simulink model "BlokSchema2"  (R2022a)
settings: Solver=VariableStepAuto  StartTime=0.0  StopTime=10000  RelTol=1e-3
undefined symbols (not defined in the file): citatel, Delay, Grz_spatnaObdlMet, Grz_tustin, menovatel, T
settings Model: PacingRate=100  Creator=domin  LastModifiedBy=domin
settings ModelReferenceCC: EnableRefExpFcnMdlSchedulingChecks=off
settings RTWCC: Description=Generic Real-Time Target

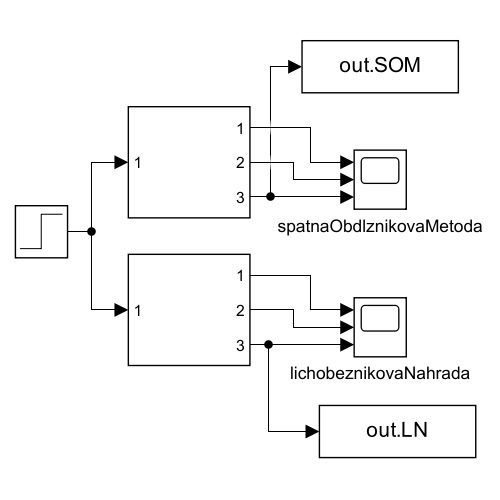
[thumbnail: Simulink's stored preview of the top-level diagram]
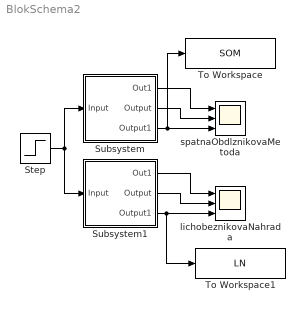
== system BlokSchema2 ==
  Step : Step  Time=0  Before=1  SampleTime=0
  Subsystem : Subsystem
  Subsystem1 : Subsystem
  To Workspace : ToWorkspace  VariableName=SOM  SampleTime=-1
  To Workspace1 : ToWorkspace  VariableName=LN  SampleTime=-1
  lichobeznikovaNahrada : Scope  NumInputPorts=3
  spatnaObdlznikovaMetoda : Scope  NumInputPorts=3
  wires:
  Step/1 -> Subsystem/1(Input), Subsystem1/1(Input)
  Subsystem/1(Out1) -> spatnaObdlznikovaMetoda/1
  Subsystem/2(Output) -> spatnaObdlznikovaMetoda/2
  Subsystem/3(Output1) -> To Workspace/1, spatnaObdlznikovaMetoda/3
  Subsystem1/1(Out1) -> lichobeznikovaNahrada/1
  Subsystem1/2(Output) -> lichobeznikovaNahrada/2
  Subsystem1/3(Output1) -> To Workspace1/1, lichobeznikovaNahrada/3

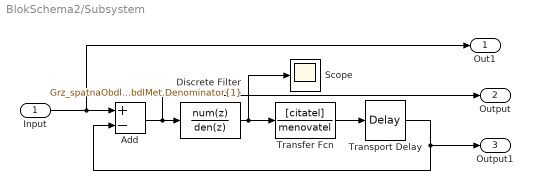
== system BlokSchema2/Subsystem ==
  Input : Inport
  Add : Sum  Inputs=+-
  Discrete Filter : DiscreteFilter  Numerator=Grz_spatnaObdlMet.Numerator{1}  Denominator=Grz_spatnaObdlMet.Denominator{1}  SampleTime=T
  Scope : Scope
  Transfer Fcn : TransferFcn  Numerator=[citatel]  Denominator=menovatel
  Transport Delay : TransportDelay  DelayTime=Delay
  Out1 : Outport
  Output : Outport  Port=2
  Output1 : Outport  Port=3
  wires:
  Add/1 -> Discrete Filter/1, Output/1
  Input/1 -> Out1/1, Add/1
  Transfer Fcn/1 -> Transport Delay/1
  Discrete Filter/1 -> Transfer Fcn/1, Scope/1
  Transport Delay/1 -> Output1/1, Add/2

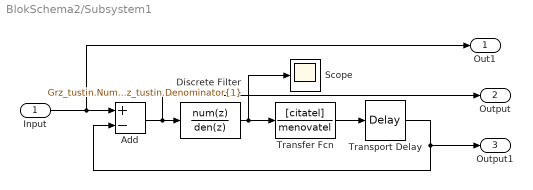
== system BlokSchema2/Subsystem1 ==
  Input : Inport
  Add : Sum  Inputs=+-
  Discrete Filter : DiscreteFilter  Numerator=Grz_tustin.Numerator{1}  Denominator=Grz_tustin.Denominator{1}  SampleTime=T
  Scope : Scope
  Transfer Fcn : TransferFcn  Numerator=[citatel]  Denominator=menovatel
  Transport Delay : TransportDelay  DelayTime=Delay
  Out1 : Outport
  Output : Outport  Port=2
  Output1 : Outport  Port=3
  wires:
  Add/1 -> Discrete Filter/1, Output/1
  Input/1 -> Out1/1, Add/1
  Transfer Fcn/1 -> Transport Delay/1
  Discrete Filter/1 -> Transfer Fcn/1, Scope/1
  Transport Delay/1 -> Output1/1, Add/2
